simulink model "HammingDecoder"  (R2020b)
settings: Solver=VariableStepAuto  StartTime=0.0  StopTime=10.0  RelTol=1e-3
settings Model: Creator=12643  LastModifiedBy=12643

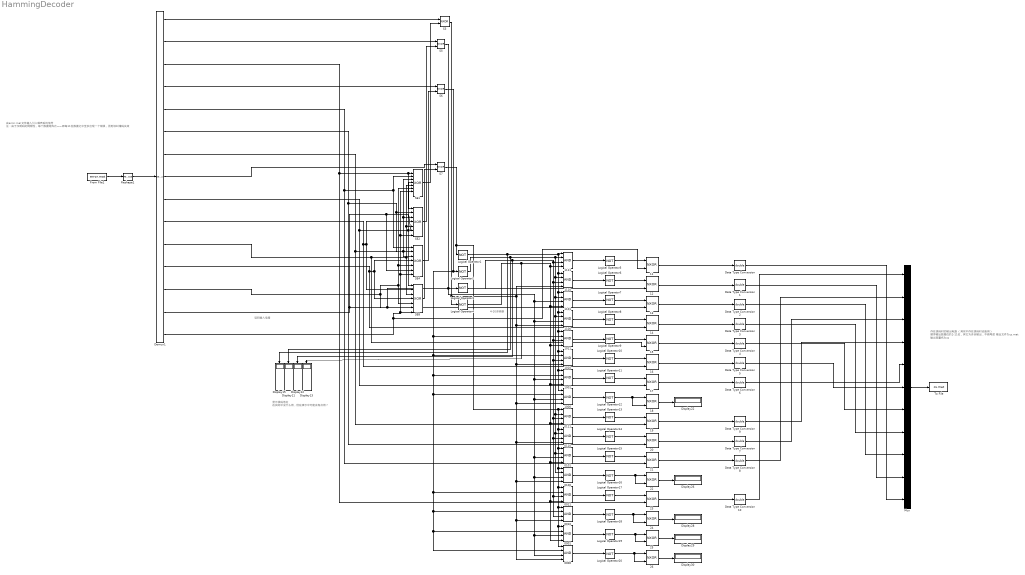
== system HammingDecoder ==
  note: 4-16译码器
  note: 误码输入电路
  note: 由error.mat文件输入引入噪声后的信号
      | 注：由于汉明码的局限性，每个数据矩阵内——即每11位数据之中至多出现一个错误，否则该纠错码失效
  note: 存在误码时的输出电路
      | （其实不存在误码时也能用）
      | 顺序输出数据位的1-11位，其它为多余输出，不做考虑
      | 输出文件为cs.mat
      | 输出变量名为cs
  note: 显示误码地址
      | 在实际中没什么用，但在演示中可能会有点用？
   {11..26} (16 alike) : Logic  Operator=NXOR  AllPortsSameDT=off  OutDataTypeStr=boolean
  0000 : Logic  Inputs=4  AllPortsSameDT=off  OutDataTypeStr=boolean
  0001 : Logic  Inputs=4  AllPortsSameDT=off  OutDataTypeStr=boolean
  0010 : Logic  Inputs=4  AllPortsSameDT=off  OutDataTypeStr=boolean
  0011 : Logic  Inputs=4  AllPortsSameDT=off  OutDataTypeStr=boolean
  0100 : Logic  Inputs=4  AllPortsSameDT=off  OutDataTypeStr=boolean
  0101 : Logic  Inputs=4  AllPortsSameDT=off  OutDataTypeStr=boolean
  0110 : Logic  Inputs=4  AllPortsSameDT=off  OutDataTypeStr=boolean
  0111 : Logic  Inputs=4  AllPortsSameDT=off  OutDataTypeStr=boolean
  {1000..1001,1010..1011,1100..1101,1110..1111} (8 alike) : Logic  Inputs=4  AllPortsSameDT=off  OutDataTypeStr=boolean
  Data Type Conversion{,1..10} (11 alike) : DataTypeConversion  OutMin=0  OutMax=1  OutDataTypeStr=double
  Demux1 : Demux  Outputs=15
  Display{11..13,15,22,26,28..30} (9 alike) : Display
  From File1 : FromFile  FileName=error.mat  SampleTime=0
  Logical Operator{1..20} (20 alike) : Logic  Operator=NOT  AllPortsSameDT=off  OutDataTypeStr=boolean
  Mux : Mux  Inputs=11
  Reshape1 : Reshape  OutputDimensionality=Customize  OutputDimensions=[15,1]
  S{3,5..7} (4 alike) : Logic  Operator=NXOR  AllPortsSameDT=off  OutDataTypeStr=boolean
  SE{1..2,4,8} (4 alike) : Logic  Operator=XOR  Inputs=7  AllPortsSameDT=off  OutDataTypeStr=boolean
  To File : ToFile  Filename=cs.mat  MatrixName=cs
  wires:
  Demux1/1 -> S3/1
  Demux1/2 -> S5/1
  Demux1/4 -> S6/1
  Demux1/8 -> S7/1
  Demux1/10 -> " 16"/2, SE8/2, SE2/4
  Demux1/9 -> " 17"/2, SE8/1, SE1/4
  Demux1/15 -> SE1/7, SE2/7, SE4/7, SE8/7, " 11"/2
  Demux1/13 -> " 13"/2, SE8/5, SE1/6, SE4/5
  Demux1/11 -> " 15"/2, SE8/3, SE1/5, SE2/5
  Demux1/12 -> " 14"/2, SE8/4, SE4/4
  Demux1/5 -> " 21"/2, SE4/1, SE1/2
  Demux1/14 -> SE2/6, SE4/6, " 12"/2, SE8/6
  Demux1/6 -> " 20"/2, SE2/2, SE4/2
  Demux1/3 -> " 23"/2, SE1/1, SE2/1
  Demux1/7 -> " 19"/2, SE1/3, SE2/3, SE4/3
  SE1/1 -> S3/2
  SE2/1 -> S5/2
  SE4/1 -> S6/2
  SE8/1 -> S7/2
  S3/1 -> 0000/4, 0010/4, 0100/4, 0110/4, 1000/4, 1010/4, 1100/4, 1110/4, Logical Operator4/1
  S5/1 -> 0000/3, 0001/3, 0100/3, 0101/3, 1000/3, 1001/3, 1100/3, 1101/3, Logical Operator3/1
  S6/1 -> 0000/2, 0001/2, 0010/2, 0011/2, 1000/2, 1001/2, 1010/2, 1011/2, Logical Operator2/1
  S7/1 -> 0000/1, 0001/1, 0010/1, 0011/1, 0100/1, 0101/1, 0110/1, 0111/1, Logical Operator1/1
  Logical Operator1/1 -> 1000/1, 1001/1, 1010/1, 1011/1, 1100/1, 1101/1, 1110/1, 1111/1, Display15/1
  Logical Operator2/1 -> Display11/1, 0100/2, 0101/2, 0110/2, 0111/2, 1100/2, 1101/2, 1110/2, 1111/2
  Logical Operator3/1 -> 0010/3, 0011/3, 0110/3, 0111/3, 1010/3, 1011/3, 1110/3, 1111/3, Display12/1
  Logical Operator4/1 -> 0001/4, 0011/4, 0101/4, 0111/4, 1001/4, 1011/4, 1101/4, 1111/4, Display13/1
  1011/1 -> Logical Operator9/1
  0000/1 -> Logical Operator20/1
  0001/1 -> Logical Operator19/1
  0010/1 -> Logical Operator18/1
  0011/1 -> Logical Operator17/1
  0100/1 -> Logical Operator16/1
  0101/1 -> Logical Operator15/1
  0110/1 -> Logical Operator14/1
  0111/1 -> Logical Operator13/1
  1000/1 -> Logical Operator12/1
  1001/1 -> Logical Operator11/1
  1010/1 -> Logical Operator10/1
  1100/1 -> Logical Operator8/1
  1101/1 -> Logical Operator7/1
  1110/1 -> Logical Operator6/1
  1111/1 -> Logical Operator5/1
  " 11"/1 -> Data Type Conversion/1
  " 12"/1 -> Data Type Conversion1/1
  " 13"/1 -> Data Type Conversion2/1
  " 14"/1 -> Data Type Conversion3/1
  " 15"/1 -> Data Type Conversion4/1
  " 16"/1 -> Data Type Conversion5/1
  " 17"/1 -> Data Type Conversion6/1
  " 18"/1 -> Display22/1
  " 19"/1 -> Data Type Conversion9/1
  " 20"/1 -> Data Type Conversion7/1
  " 21"/1 -> Data Type Conversion8/1
  " 22"/1 -> Display26/1
  " 23"/1 -> Data Type Conversion10/1
  " 24"/1 -> Display28/1
  " 25"/1 -> Display29/1
  " 26"/1 -> Display30/1
  Logical Operator17/1 -> " 23"/1
  Logical Operator18/1 -> " 24"/2, " 24"/1
  Logical Operator19/1 -> " 25"/2, " 25"/1
  Logical Operator20/1 -> " 26"/2, " 26"/1
  Logical Operator16/1 -> " 22"/2, " 22"/1
  Logical Operator15/1 -> " 21"/1
  Logical Operator14/1 -> " 20"/1
  Logical Operator13/1 -> " 19"/1
  Logical Operator12/1 -> " 18"/2, " 18"/1
  Logical Operator11/1 -> " 17"/1
  Logical Operator10/1 -> " 16"/1
  Logical Operator9/1 -> " 15"/1
  Logical Operator8/1 -> " 14"/1
  Logical Operator7/1 -> " 13"/1
  Logical Operator6/1 -> " 12"/1
  Logical Operator5/1 -> " 11"/1
  Mux/1 -> To File/1
  Reshape1/1 -> Demux1/1
  From File1/1 -> Reshape1/1
  Data Type Conversion10/1 -> Mux/1
  Data Type Conversion8/1 -> Mux/2
  Data Type Conversion7/1 -> Mux/3
  Data Type Conversion9/1 -> Mux/4
  Data Type Conversion6/1 -> Mux/5
  Data Type Conversion5/1 -> Mux/6
  Data Type Conversion4/1 -> Mux/7
  Data Type Conversion3/1 -> Mux/8
  Data Type Conversion2/1 -> Mux/9
  Data Type Conversion1/1 -> Mux/10
  Data Type Conversion/1 -> Mux/11
